simulink model "PTC_MBDS_IntegratorT_REL_Sample"  (R2013a)
settings: Solver=FixedStepDiscrete  StartTime=0.0  StopTime=100  FixedStep=Auto  RelTol=1e-3
undefined symbols (not defined in the file): sigbuilder_block
libraries: simulink_extras x1, PTC_MBDS_LIB x1
settings Model: Creator=uidl7367  LastModifiedBy=sundeep.tuteja
settings DataIOCC: SignalLoggingSaveFormat=ModelDataLogs
settings OptimizationCC: ExpressionDepthLimit=2147483647  InitFltsAndDblsToZero=on
settings DebuggingCC: SaveWithParameterizedLinksMsg=none  SignalResolutionControl=TryResolveAllWithWarning  SolverPrmCheckMsg=none  InheritedTsInSrcMsg=none  MultiTaskDSMMsg=warning  MultiTaskCondExecSysMsg=none  FcnCallInpInsideContextMsg=UseLocalSettings  StrictBusMsg=Warning
settings RTWCC: IncludeERTFirstTime=on
settings GRTTargetCC: TargetFcnLib=ansi_tfl_tmw.mat  CombineOutputUpdateFcns=off  GRTInterface=on

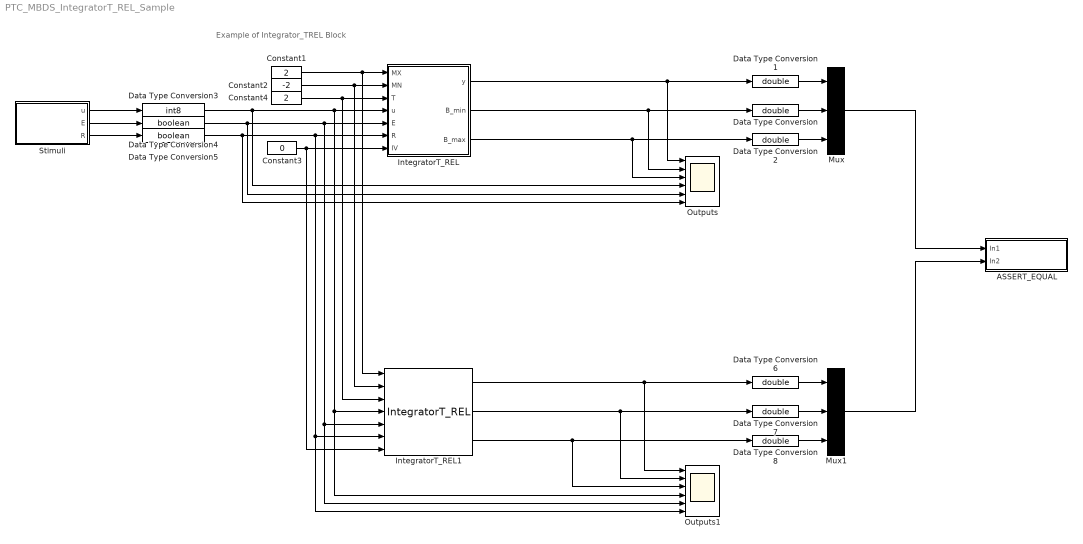
== system PTC_MBDS_IntegratorT_REL_Sample ==
  note: Example of Integrator_TREL Block
  ASSERT_EQUAL : Subsystem
  Constant1 : Constant  InitFcn=|  Value=2  VectorParams1D=off  OutDataTypeStr=Inherit: Inherit via back propagation
      | if(exist('MBDS_BlockCallback', 'file'))
      |    MBDS_BlockCallback('Update', gcb);  
      | end
  Constant2 : Constant  InitFcn=|  Value=-2  VectorParams1D=off  OutDataTypeStr=int8
      | if(exist('MBDS_BlockCallback', 'file'))
      |    MBDS_BlockCallback('Update', gcb);  
      | end
  Constant3 : Constant  InitFcn=|  Value=0  VectorParams1D=off  OutDataTypeStr=Inherit: Inherit via back propagation
      | if(exist('MBDS_BlockCallback', 'file'))
      |    MBDS_BlockCallback('Update', gcb);  
      | end
  Constant4 : Constant  InitFcn=|  Value=2  VectorParams1D=off  OutDataTypeStr=Inherit: Inherit via back propagation
      | if(exist('MBDS_BlockCallback', 'file'))
      |    MBDS_BlockCallback('Update', gcb);  
      | end
  Data Type Conversion3 : DataTypeConversion  InitFcn=|  OutDataTypeStr=int8  SaturateOnIntegerOverflow=on
      | try
      |    MBDS_BlockCallback('Update', gcb);
      | end
  Data Type Conversion4 : DataTypeConversion  InitFcn=|  OutDataTypeStr=boolean  SaturateOnIntegerOverflow=on
      | try
      |    MBDS_BlockCallback('Update', gcb);
      | end
  Data Type Conversion5 : DataTypeConversion  InitFcn=|  OutDataTypeStr=boolean  SaturateOnIntegerOverflow=on
      | try
      |    MBDS_BlockCallback('Update', gcb);
      | end
  Data Type Conversion{,1..2,6..8} (6 alike) : DataTypeConversion  OutDataTypeStr=double
  IntegratorT_REL : Subsystem  InitFcn=|  mask(IntegratorT_REL){MBDS_LibraryBlock=on, MXMN_Enabled=on, MX=0, MN=0, dT_Enabled=off, dT=1, E_Enabled=on, R_Enabled=on, IV_Enabled=on, IV=0, B_min_Enabled=on, B_max_Enabled=on, MBDS_BlockVersion=05.40}
      | if(exist('MBDS_BlockCallback', 'file'))
      |    MBDS_BlockCallback('Update', gcb);
      | end
      mask prompts: MBDS_LibraryBlock "MBDS library block"; MXMN_Enabled "Show MX/MN port"; MX "Upper limit (MX):"; MN "Lower limit (MN):"; dT_Enabled "Show dT port"; dT "Sample rate (dT):"; E_Enabled "Show E port"; R_Enabled "Show R port"; IV_Enabled "Show IV port"; IV "Initial value (IV):"; B_min_Enabled "Show B_min port"; B_max_Enabled "Show B_max port"; MBDS_BlockVersion "Block version:"
      mask help: A time discrete integrator with gain 1/T and limitation of the integrator value y to the maximum MX and the minimum MN.
      mask init:
      | if(exist('MBDS_BlockCallback', 'file'))
      |    MBDS_BlockCallback('Init', gcb);
      | else
      |    % Disable all mask parameters
      |    MaskEnables = get_param(gcb, 'MaskEnables');
      |    for k = [1:length(MaskEnables)]
      |       MaskEnables{k} = 'off';
      |    end
      |    if(~isequal(MaskEnables, get_param(gcb, 'MaskEnables')))
      |       set_param(gcb, 'MaskEnables', MaskEnables);
      |    end
      | end
      settings: AttributesFormatString=dT = %<dT>
      mask Help: eval(['open([workdir(''library_dir:''),''\Blockset\help\'',get_param(gcb,''MaskType''),''.html''])'])
      mask Callback MXMN_Enabled:
      | % Update mask parameter dialog
      | if(exist('MBDS_BlockCallback', 'file'))
      |    MBDS_BlockCallback('MXMN_Enabled', gcb);
      | end
      mask Callback MX:
      | % Adopt Value
      | if(exist('MBDS_BlockCallback', 'file'))
      |    MBDS_BlockCallback('MX', gcb);
      | end
      mask Callback MN:
      | % Adopt Value
      | if(exist('MBDS_BlockCallback', 'file'))
      |    MBDS_BlockCallback('MN', gcb);
      | end
      mask Callback dT_Enabled:
      | % Update mask parameter dialog
      | if(exist('MBDS_BlockCallback', 'file'))
      |    MBDS_BlockCallback('dT_Enabled', gcb);
      | end
      mask Callback dT:
      | % Adopt Value
      | if(exist('MBDS_BlockCallback', 'file'))
      |    MBDS_BlockCallback('dT', gcb);
      | end
      mask Callback R_Enabled:
      | % Update mask parameter dialog
      | if(exist('MBDS_BlockCallback', 'file'))
      |    MBDS_BlockCallback('R_Enabled', gcb);
      | end
      mask Callback IV_Enabled:
      | % Update mask parameter dialog
      | if(exist('MBDS_BlockCallback', 'file'))
      |    MBDS_BlockCallback('IV_Enabled', gcb);
      | end
      mask Callback IV:
      | % Adopt Value
      | if(exist('MBDS_BlockCallback', 'file'))
      |    MBDS_BlockCallback('IV', gcb);
      | end
      mask Callback B_min_Enabled:
      | % Update mask parameter dialog
      | if(exist('MBDS_BlockCallback', 'file'))
      |    MBDS_BlockCallback('B_min_Enabled', gcb);
      | end
      mask Callback B_max_Enabled:
      | % Update mask parameter dialog
      | if(exist('MBDS_BlockCallback', 'file'))
      |    MBDS_BlockCallback('B_max_Enabled', gcb);
      | end
      mask Display:
      | % Show icon or block text
      | if(exist('IntegratorT.tif', 'file'))
      |    image(imread('IntegratorT.tif','tif'), [0.248421052631579 0.342857142857143 0.378947368421053 0.314285714285714]);
      |    disp('')
      | else
      |    disp(sprintf('Integrator\n\n'));
      | end
      | 
      | % Display port labels
      | port_label('input', 1, 'MX');
      | port_label('input', 2, 'MN');
      | port_label('input', 3, 'T');
      | port_label('input', 4, 'u');
      | port_label('input', 5, 'E');
      | port_label('input', 6, 'R');
      | port_label('input', 7, 'IV');
      | port_label('output', 1, 'y');
      | port_label('output', 2, 'B_min');
      | port_label('output', 3, 'B_max');
  IntegratorT_REL1 : PTC_MBDS_LIB/MBDS Standard Library/Extended Operations/Integrators/IntegratorT_REL  MXMN_Enabled=on  MX=0  MN=0  dT_Enabled=off  dT=1  E_Enabled=on  R_Enabled=on  IV_Enabled=on  IV=0  B_min_Enabled=on  B_max_Enabled=on  PTC_MBDS_BlockVersion=5.32  PTC_BlockType=PTC_MBDS_IntegratorT_REL
      settings: AttributesFormatString=dT = %<dT>
  Mux : Mux  Inputs=3
  Mux1 : Mux  Inputs=3
  Outputs : Scope  NumInputPorts=6
      settings: TimeRange=100  YMin=-2~0~0~-2~0~0  YMax=2~1~1~4~1~1  SampleInput=on  SampleTime=1
  Outputs1 : Scope  NumInputPorts=6
      settings: TimeRange=100  YMin=-2~0~0~-2~0~0  YMax=2~1~1~4~1~1  SampleInput=on  SampleTime=1
  Stimuli : Subsystem  Tag=STV Subsys  LoadFcn=sigbuilder_block('load');  StartFcn=sigbuilder_block('start');  StopFcn=sigbuilder_block('stop');  ClipboardFcn=sigbuilder_block('clipboard');  mask(Sigbuilder block){}
      mask help: Sigbuilder GUI
      mask init:
      | if ~strcmp(get_param(bdroot(gcb),'SimulationStatus'),'stopped') tuvar = sigbuilder_block('maskInit'); end
      settings: CopyFcn=sigbuilder_block('copy');  DeleteFcn=sigbuilder_block('delete');  ModelCloseFcn=sigbuilder_block('modelClose');  PreSaveFcn=sigbuilder_block('preSave');  PauseFcn=sigbuilder_block('pause')  ContinueFcn=sigbuilder_block('continue')  NameChangeFcn=sigbuilder_block('namechange');  OpenFcn=sigbuilder_block('open',[19.5 203.25 730.5 304.5 ]);  CloseFcn=sigbuilder_block('close');
      mask Display: plot(0,0,100,100,[10,10,40,40,10],[80,20,20,80,80],[40,10],[50,50], [40,27,10],[65,72,56],[40,25,25,10],[28,28,43,43]);
  wires:
  Stimuli/1(u) -> Data Type Conversion3/1
  Stimuli/2(E) -> Data Type Conversion4/1
  Stimuli/3(R) -> Data Type Conversion5/1
  IntegratorT_REL/1(y) -> Data Type Conversion1/1, Outputs/1
  IntegratorT_REL/2(B_min) -> Data Type Conversion/1, Outputs/2
  IntegratorT_REL/3(B_max) -> Outputs/3, Data Type Conversion2/1
  Constant1/1 -> IntegratorT_REL/1(MX), IntegratorT_REL1/1
  Constant2/1 -> IntegratorT_REL/2(MN), IntegratorT_REL1/2
  Constant4/1 -> IntegratorT_REL/3(T), IntegratorT_REL1/3
  Data Type Conversion3/1 -> IntegratorT_REL/4(u), Outputs1/4, IntegratorT_REL1/4, Outputs/4
  Data Type Conversion4/1 -> IntegratorT_REL/5(E), Outputs1/5, IntegratorT_REL1/5, Outputs/5
  Data Type Conversion5/1 -> IntegratorT_REL/6(R), Outputs1/6, IntegratorT_REL1/6, Outputs/6
  Constant3/1 -> IntegratorT_REL/7(IV), IntegratorT_REL1/7
  IntegratorT_REL1/3 -> Data Type Conversion8/1, Outputs1/3
  IntegratorT_REL1/2 -> Outputs1/2, Data Type Conversion7/1
  IntegratorT_REL1/1 -> Data Type Conversion6/1, Outputs1/1
  Mux/1 -> ASSERT_EQUAL/1(In1)
  Mux1/1 -> ASSERT_EQUAL/2(In2)
  Data Type Conversion1/1 -> Mux/1
  Data Type Conversion/1 -> Mux/2
  Data Type Conversion2/1 -> Mux/3
  Data Type Conversion6/1 -> Mux1/1
  Data Type Conversion7/1 -> Mux1/2
  Data Type Conversion8/1 -> Mux1/3

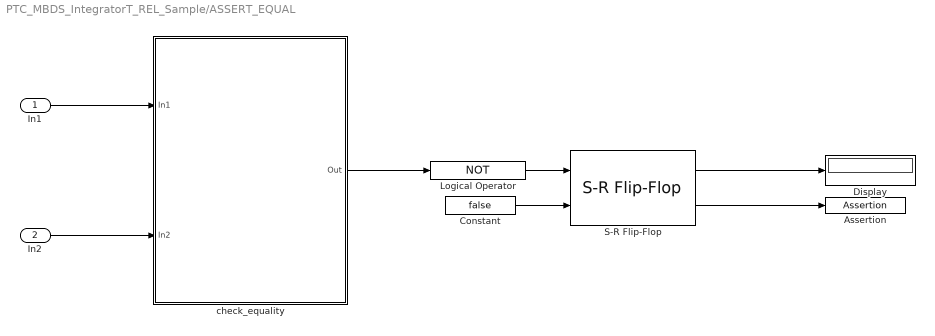
== system PTC_MBDS_IntegratorT_REL_Sample/ASSERT_EQUAL ==
  In1 : Inport
  In2 : Inport  Port=2
  Assertion : Assertion
  Constant : Constant  Value=false
  Display : Display
  Logical Operator : Logic  Operator=NOT  AllPortsSameDT=off  OutDataTypeStr=boolean
  S-R Flip-Flop : simulink_extras/Flip Flops/S-R Flip-Flop  initial_condition=0
  check_equality : MATLAB Function  TreatAsAtomicUnit=on
  wires:
  S-R Flip-Flop/1 -> Display/1
  check_equality/1(Out) -> Logical Operator/1
  Constant/1 -> S-R Flip-Flop/2
  S-R Flip-Flop/2 -> Assertion/1
  In2/1 -> check_equality/2(In2)
  In1/1 -> check_equality/1(In1)
  Logical Operator/1 -> S-R Flip-Flop/1

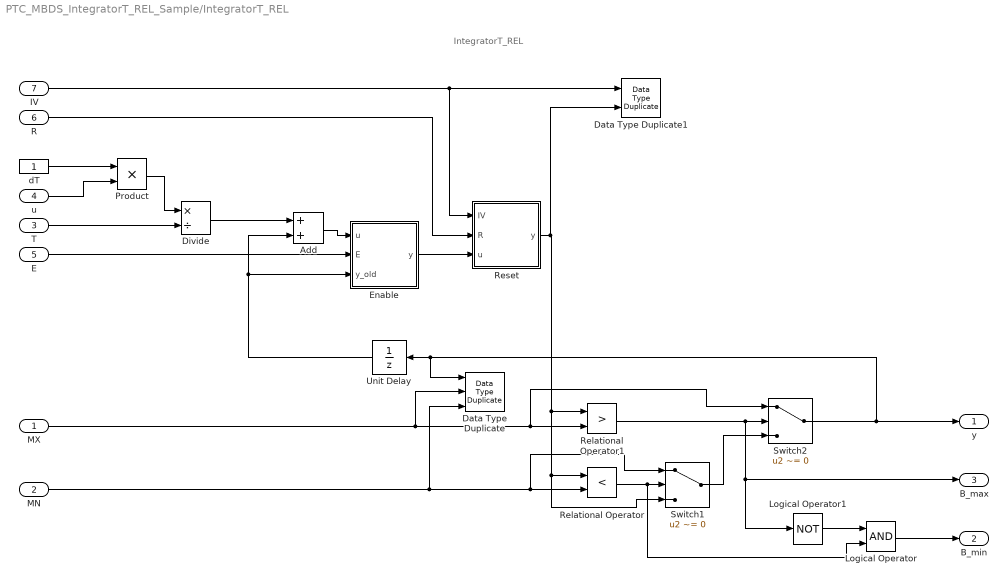
== system PTC_MBDS_IntegratorT_REL_Sample/IntegratorT_REL ==
  note: IntegratorT_REL
  MX : Inport
  MN : Inport  Port=2
  T : Inport  Port=3
  u : Inport  Port=4
  E : Inport  Port=5  OutDataTypeStr=boolean
  R : Inport  Port=6  OutDataTypeStr=boolean
  IV : Inport  Port=7
  Add : Sum  OutDataTypeStr=Inherit: Inherit via back propagation  SaturateOnIntegerOverflow=on
  Data Type Duplicate : DataTypeDuplicate  NumInputPorts=3
  Data Type Duplicate1 : DataTypeDuplicate
  Divide : Product  Inputs=*/
  Enable : Subsystem
  Logical Operator : Logic  AllPortsSameDT=off  OutDataTypeStr=boolean
  Logical Operator1 : Logic  Operator=NOT  AllPortsSameDT=off  OutDataTypeStr=boolean
  Product : Product
  Relational Operator : RelationalOperator  Operator=<  OutDataTypeStr=boolean
  Relational Operator1 : RelationalOperator  Operator=>  OutDataTypeStr=boolean
  Reset : Subsystem
  Switch1 : Switch  Criteria=u2 ~= 0  OutDataTypeStr=Inherit: Inherit via back propagation  SaturateOnIntegerOverflow=on
  Switch2 : Switch  Criteria=u2 ~= 0  OutDataTypeStr=Inherit: Inherit via back propagation  SaturateOnIntegerOverflow=on
  Unit Delay : UnitDelay  SampleTime=-1
  dT : Constant  OutDataTypeStr=Inherit: Inherit via back propagation
  y : Outport
  B_min : Outport  Port=2
  B_max : Outport  Port=3
  wires:
  dT/1 -> Product/1
  u/1 -> Product/2
  Unit Delay/1 -> Enable/3(y_old), Add/2
  Add/1 -> Enable/1(u)
  IV/1 -> Reset/1(IV), Data Type Duplicate1/1
  Enable/1(y) -> Reset/3(u)
  Switch2/1 -> y/1, Unit Delay/1, Data Type Duplicate/1
  Switch1/1 -> Switch2/3
  Relational Operator/1 -> Logical Operator/2, Switch1/2
  Relational Operator1/1 -> Switch2/2, B_max/1, Logical Operator1/1
  MN/1 -> Switch1/1, Relational Operator/2, Data Type Duplicate/3
  Logical Operator1/1 -> Logical Operator/1
  Logical Operator/1 -> B_min/1
  Reset/1(y) -> Data Type Duplicate1/2, Relational Operator/1, Switch1/3, Relational Operator1/1
  MX/1 -> Data Type Duplicate/2, Switch2/1, Relational Operator1/2
  Divide/1 -> Add/1
  T/1 -> Divide/2
  Product/1 -> Divide/1
  R/1 -> Reset/2(R)
  E/1 -> Enable/2(E)

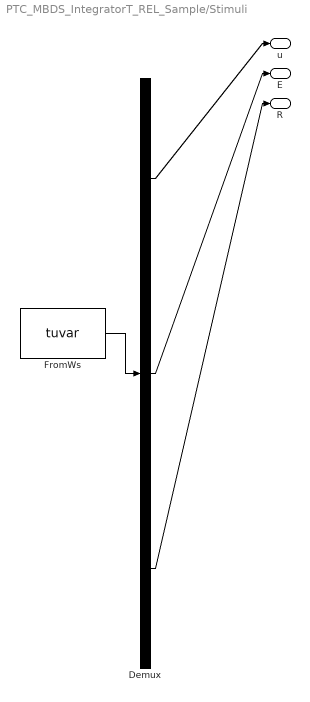
== system PTC_MBDS_IntegratorT_REL_Sample/Stimuli ==
  Demux : Demux  Tag=STV Demux  Outputs=3
  FromWs : FromWorkspace  Tag=STV FromWs  VariableName=tuvar  OutputAfterFinalValue=Holding final value
      SigBuilderData=|
      | common.afterFinalStr = 'Hold final value'
      | common.sampleTime = -1
      | dataSet.timeRange = [0 100]
      | dataSet.name = 'test data'
      | sbobj.Groups.Name = 'test data'
      | sbobj.Groups.Signals(1).Name = 'u'
      | sbobj.Groups.Signals(1).XData = [0 50 50 70 70 100]
      | sbobj.Groups.Signals(1).YData = [1 1 3 3 -2 -2]
      | sbobj.Groups.Signals(2).Name = 'E'
      | sbobj.Groups.Signals(2).XData = [0 10 10 20 20 100]
      | sbobj.Groups.Signals(2).YData = [1 1 0 0 1 1]
      | sbobj.Groups.Signals(3).Name = 'R'
      | sbobj.Groups.Signals(3).XData = [0 29.5 29.5 30.5 30.5 100]
      | sbobj.Groups.Signals(3).YData = [0 0 1 1 0 0]
      | sbobj.Groups.TimeRange = [0 100]
  u : Outport  Tag=STV Outport
  E : Outport  Tag=STV Outport  Port=2
  R : Outport  Tag=STV Outport  Port=3
  wires:
  Demux/3 -> R/1
  Demux/2 -> E/1
  Demux/1 -> u/1
  FromWs/1 -> Demux/1

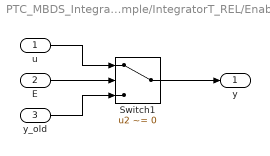
== system PTC_MBDS_IntegratorT_REL_Sample/IntegratorT_REL/Enable ==
  u : Inport
  E : Inport  Port=2
  y_old : Inport  Port=3
  Switch1 : Switch  Criteria=u2 ~= 0  OutDataTypeStr=Inherit: Inherit via back propagation  InputSameDT=on
  y : Outport
  wires:
  E/1 -> Switch1/2
  u/1 -> Switch1/1
  Switch1/1 -> y/1
  y_old/1 -> Switch1/3

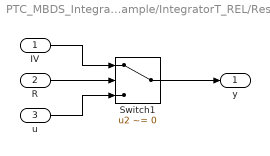
== system PTC_MBDS_IntegratorT_REL_Sample/IntegratorT_REL/Reset ==
  IV : Inport
  R : Inport  Port=2
  u : Inport  Port=3
  Switch1 : Switch  Criteria=u2 ~= 0  OutDataTypeStr=Inherit: Inherit via back propagation  InputSameDT=on
  y : Outport
  wires:
  R/1 -> Switch1/2
  IV/1 -> Switch1/1
  Switch1/1 -> y/1
  u/1 -> Switch1/3

== matlab function PTC_MBDS_IntegratorT_REL_Sample/ASSERT_EQUAL/check_equality ==
  data: In1 input; Out output; In2 input
function Out = check_equality(In1, In2)
%#codegen

Out = isequaln(In1, In2);

end
